simulink model "sync_flier_modelling_non_d_no_spring"  (R2021a)
settings: Solver=FixedStepAuto  StartTime=0.0  StopTime=500  FixedStep=dt  RelTol=1e-3
values from neighbouring files (symbols this model uses):
  P1 = P1allnew(1,p1i)    [Find_Lambda_F_by_K_diff_amp_async.m]    (also in Find_Lamda_F_by_K_async.m; Find_Lamda_F_by_K_sync.m = P1allfinal(1,p1i); Find_Lamda_F_by_K_sync_no_spring.m = P1allfinal(1,p1i))
  P2 = P2 + limitasync(p1i,1)    [Find_Lambda_F_by_K_diff_amp_async.m]    (also in Find_Lamda_F_by_K_async.m = 0.1; Find_Lamda_F_by_K_sync.m = P2new(1,p1i); Find_Lamda_F_by_K_sync_no_spring.m = P2new(1,p1i))
  P3 = P3all(p3i)    [Find_Lamda_F_by_K_sync.m]    (also in Find_Lamda_F_by_K_sync_no_spring.m)
libraries: simulink x2
settings Model: Creator=suyash  LastModifiedBy=suyash
settings SolverCC: ZeroCrossAlgorithm=Adaptive

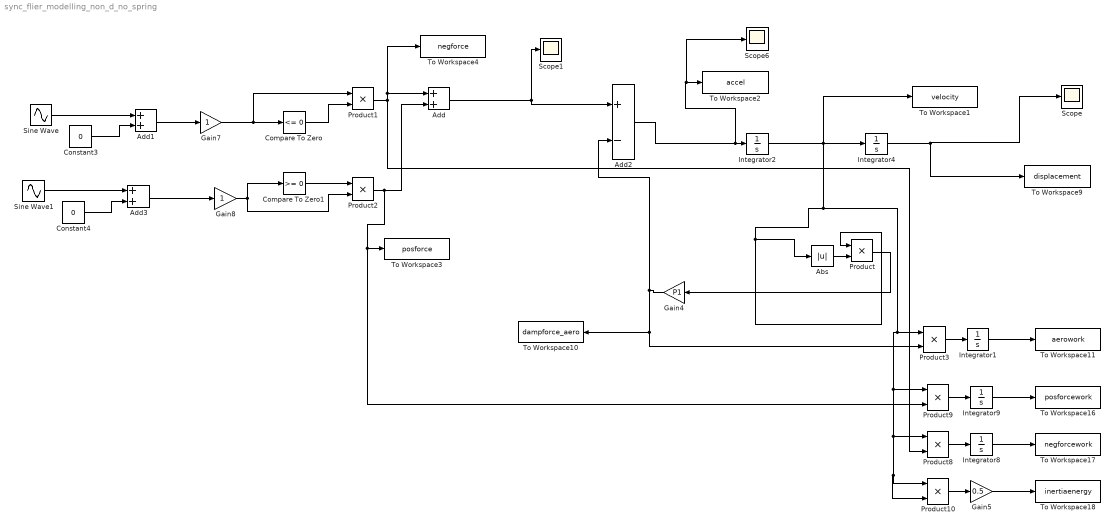
== system sync_flier_modelling_non_d_no_spring ==
  Abs : Abs
  Add : Sum
  Add1 : Sum
  Add2 : Sum  Inputs=+-
  Add3 : Sum
  Compare To Zero : simulink/Logic and Bit Operations/Compare To Zero  relop=<=  OutDataTypeStr=boolean
  Compare To Zero1 : simulink/Logic and Bit Operations/Compare To Zero  relop=>=  OutDataTypeStr=boolean
  Constant3 : Constant  Value=0
  Constant4 : Constant  Value=0
  Gain4 : Gain  Gain=P1
  Gain5 : Gain  Gain=0.5
  Gain7 : Gain
  Gain8 : Gain
  Integrator{1..2,4,8..9} (5 alike) : Integrator
  Product{,1..3,8..10} (7 alike) : Product
  Scope : Scope
  Scope1 : Scope
  Scope6 : Scope
  Sine Wave : Sin  Amplitude=P2  Frequency=P3  SampleTime=0
  Sine Wave1 : Sin  Amplitude=P2  Frequency=P3  SampleTime=0
  To Workspace1 : ToWorkspace  VariableName=velocity  SaveFormat=Timeseries  SampleTime=-1
  To Workspace10 : ToWorkspace  VariableName=dampforce_aero  SaveFormat=Timeseries  SampleTime=-1
  To Workspace11 : ToWorkspace  VariableName=aerowork  SaveFormat=Timeseries  SampleTime=-1
  To Workspace16 : ToWorkspace  VariableName=posforcework  SaveFormat=Timeseries  SampleTime=-1
  To Workspace17 : ToWorkspace  VariableName=negforcework  SaveFormat=Timeseries  SampleTime=-1
  To Workspace18 : ToWorkspace  VariableName=inertiaenergy  SaveFormat=Timeseries  SampleTime=-1
  To Workspace2 : ToWorkspace  VariableName=accel  SaveFormat=Timeseries  SampleTime=-1
  To Workspace3 : ToWorkspace  VariableName=posforce  SaveFormat=Timeseries  SampleTime=-1
  To Workspace4 : ToWorkspace  VariableName=negforce  SaveFormat=Timeseries  SampleTime=-1
  To Workspace9 : ToWorkspace  VariableName=displacement  SaveFormat=Timeseries  SampleTime=-1
  wires:
  Product/1 -> Gain4/1
  Abs/1 -> Product/2
  Integrator9/1 -> To Workspace16/1
  Gain4/1 -> Add2/2, Product3/2, To Workspace10/1
  Integrator8/1 -> To Workspace17/1
  Product8/1 -> Integrator8/1
  Product9/1 -> Integrator9/1
  Integrator1/1 -> To Workspace11/1
  Product10/1 -> Gain5/1
  Product3/1 -> Integrator1/1
  Gain5/1 -> To Workspace18/1
  Add2/1 -> Scope6/1, To Workspace2/1, Integrator2/1
  Gain7/1 -> Compare To Zero/1, Product1/1
  Gain8/1 -> Product2/2, Compare To Zero1/1
  Constant3/1 -> Add1/2
  Sine Wave/1 -> Add1/1
  Add1/1 -> Gain7/1
  Product2/1 -> Product9/2, To Workspace3/1, Add/2
  Product1/1 -> To Workspace4/1, Add/1, Product8/2
  Add3/1 -> Gain8/1
  Sine Wave1/1 -> Add3/1
  Constant4/1 -> Add3/2
  Compare To Zero/1 -> Product1/2
  Compare To Zero1/1 -> Product2/1
  Integrator2/1 -> To Workspace1/1, Integrator4/1, Product/1, Abs/1, Product10/2, Product10/1, Product8/1, Product9/1, Product3/1
  Integrator4/1 -> Scope/1, To Workspace9/1
  Add/1 -> Scope1/1, Add2/1
